simulink model "LyRStEnCtrl"  (R2018b)
settings: Solver=FixedStepDiscrete  StartTime=0.0  StopTime=10.0  FixedStep=0.01  RelTol=1e-3
undefined symbols (not defined in the file or in its folder): data, KeSMSw4SSecRwRtStLgrstUpwdDnwdOpenPos1_Val, SecRwRtStBkReclnEn_Clear, SecRwRtStBkReclnEn_Set, SecRwRtStFtrstEn_Clear, SecRwRtStFtrstEn_Set, SecRwRtStFwdBkwdEn_Clear, SecRwRtStFwdBkwdEn_Set, SecRwRtStHdrstFwdBkwdEn_Clear, SecRwRtStHdrstFwdBkwdEn_Set, SecRwRtStHdrstUpwdDnwdEn_Clear, SecRwRtStHdrstUpwdDnwdEn_Set, SecRwRtStLgrstInwdOtwdEn_Clear, SecRwRtStLgrstInwdOtwdEn_Set, SecRwRtStLgrstUpwdDnwdEn_Clear, SecRwRtStLgrstUpwdDnwdEn_Set
libraries: simulink x16
settings Model: ModifiedHistory="2023.11.16  V2.3.0 Issue 566045 全躺，vip，腿托打开增加前后位置"  Creator=sn2xws  LastModifiedBy=sn2xws
settings DataIOCC: SaveFormat=StructureWithTime
settings OptimizationCC: DefaultParameterBehavior=Inlined  EnhancedBackFolding=on  PassReuseOutputArgsAs=Individual arguments  ZeroExternalMemoryAtStartup=off  ZeroInternalMemoryAtStartup=off  OptimizeBlockOrder=speed  DifferentSizesBufferReuse=on  OptimizationCustomize=off
settings DebuggingCC: ParameterTunabilityLossMsg=error
settings ModelReferenceCC: ModelReferenceNumInstancesAllowed=Single
settings SFSimCC: MATLABDynamicMemAlloc=off
settings RTWCC: SystemTargetFile=autosar.tlc  GenCodeOnly=on  TemplateMakefile=ert_default_tmf  Description=AUTOSAR  GenerateReport=on  IncludeHyperlinkInReport=on  LaunchReport=on  GenerateTraceInfo=on  GenerateTraceReport=on  GenerateTraceReportSl=on  GenerateTraceReportSf=on  GenerateTraceReportEml=on
settings CodeAppCC: ForceParamTrailComments=on  IgnoreCustomStorageClasses=off  OperatorAnnotations=on  SimulinkDataObjDesc=on  SFDataObjDesc=on  InsertBlockDesc=on
settings STFCustomTargetCC: TargetLangStandard=C99 (ISO)  MultiwordLength=256  ParMdlRefBuildCompliant=on  CompOptLevelCompliant=on  IncludeMdlTerminateFcn=off  CombineOutputUpdateFcns=on  SuppressErrorStatus=on  ERTCustomFileBanners=on  SupportNonFinite=off  SupportComplex=off  SupportContinuousTime=off  SupportNonInlinedSFcns=off  RemoveResetFunc=on  MATLABClassNameForMDSCustomization=Simulink.SoftwareTarget.ERTCustomization  AutosarCompliant=on  UseToolchainInfoCompliant=on  LookupTableObjectStructAxisOrder=2,1,3,4,...  LUTObjectStructOrderEvenSpacing=Size,Table,Breakpoints  SystemTargetFile=autosar.tlc
settings ERTTargetCC: TargetLangStandard=C99 (ISO)  ConcurrentExecutionCompliant=off  IncludeMdlTerminateFcn=off  SuppressErrorStatus=on  SupportNonFinite=off  SupportComplex=off  ModelStepFunctionPrototypeControlCompliant=off  CPPClassGenCompliant=off  AutosarCompliant=on  LookupTableObjectStructAxisOrder=2,1,3,4,...  LUTObjectStructOrderEvenSpacing=Size,Table,Breakpoints  InlinedParameterPlacement=NonHierarchical  ERTCustomFileTemplate=example_file_process.tlc  ERTFilePackagingFormat=Compact

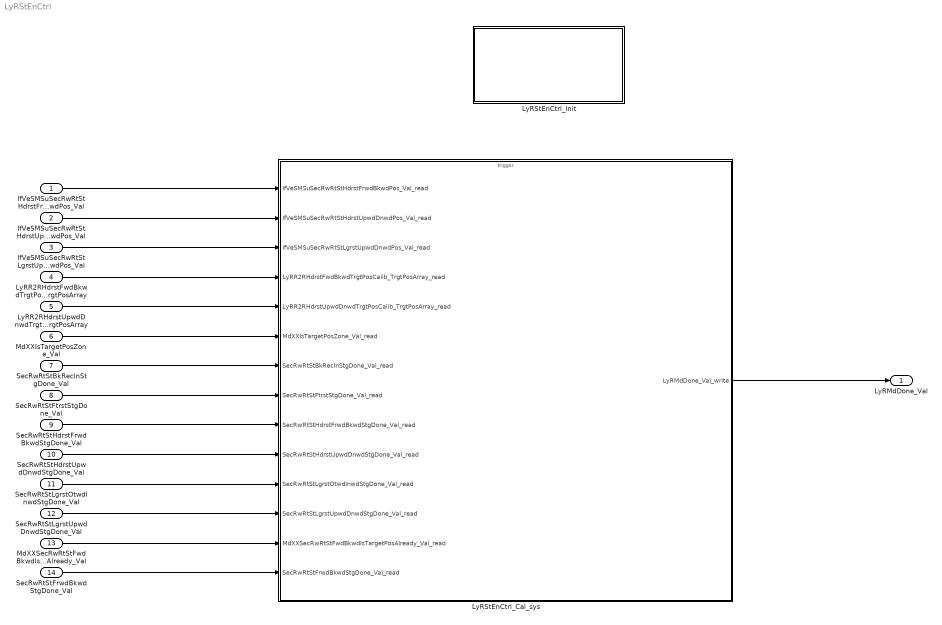
== system LyRStEnCtrl ==
  IfVeSMSuSecRwRtStHdrstFrwdBkwdPos_Val : Inport  OutDataTypeStr=uint16  PortDimensions=1
  IfVeSMSuSecRwRtStHdrstUpwdDnwdPos_Val : Inport  Port=2  OutDataTypeStr=uint16  PortDimensions=1
  IfVeSMSuSecRwRtStLgrstUpwdDnwdPos_Val : Inport  Port=3  OutDataTypeStr=uint16  PortDimensions=1
  LyRR2RHdrstFwdBkwdTrgtPosCalib_TrgtPosArray : Inport  Description=|  Port=4  OutDataTypeStr=uint16  PortDimensions=3
      | 0:Pos
      | 1:Max
      | 2:Min
  LyRR2RHdrstUpwdDnwdTrgtPosCalib_TrgtPosArray : Inport  Description=|  Port=5  OutDataTypeStr=uint16  PortDimensions=3
      | 0:Pos
      | 1:Max
      | 2:Min
  MdXXIsTargetPosZone_Val : Inport  Port=6  OutDataTypeStr=uint32  PortDimensions=1
  SecRwRtStBkReclnStgDone_Val : Inport  Port=7  OutDataTypeStr=boolean  PortDimensions=1
  SecRwRtStFtrstStgDone_Val : Inport  Port=8  OutDataTypeStr=boolean  PortDimensions=1
  SecRwRtStHdrstFrwdBkwdStgDone_Val : Inport  Port=9  OutDataTypeStr=boolean  PortDimensions=1
  SecRwRtStHdrstUpwdDnwdStgDone_Val : Inport  Port=10  OutDataTypeStr=boolean  PortDimensions=1
  SecRwRtStLgrstOtwdInwdStgDone_Val : Inport  Port=11  OutDataTypeStr=boolean  PortDimensions=1
  SecRwRtStLgrstUpwdDnwdStgDone_Val : Inport  Port=12  OutDataTypeStr=boolean  PortDimensions=1
  MdXXSecRwRtStFwdBkwdIsTargetPosAlready_Val : Inport  Port=13  OutDataTypeStr=uint32  PortDimensions=1
  SecRwRtStFrwdBkwdStgDone_Val : Inport  Port=14  OutDataTypeStr=boolean  PortDimensions=1
  LyRStEnCtrl_Cal_sys : Subsystem
  LyRStEnCtrl_Init : Subsystem
  LyRMdDone_Val : Outport  OutDataTypeStr=uint8  PortDimensions=1
  wires:
  IfVeSMSuSecRwRtStHdrstFrwdBkwdPos_Val/1 -> LyRStEnCtrl_Cal_sys/1(IfVeSMSuSecRwRtStHdrstFrwdBkwdPos_Val_read)
  IfVeSMSuSecRwRtStHdrstUpwdDnwdPos_Val/1 -> LyRStEnCtrl_Cal_sys/2(IfVeSMSuSecRwRtStHdrstUpwdDnwdPos_Val_read)
  IfVeSMSuSecRwRtStLgrstUpwdDnwdPos_Val/1 -> LyRStEnCtrl_Cal_sys/3(IfVeSMSuSecRwRtStLgrstUpwdDnwdPos_Val_read)
  LyRR2RHdrstFwdBkwdTrgtPosCalib_TrgtPosArray/1 -> LyRStEnCtrl_Cal_sys/4(LyRR2RHdrstFwdBkwdTrgtPosCalib_TrgtPosArray_read)
  LyRR2RHdrstUpwdDnwdTrgtPosCalib_TrgtPosArray/1 -> LyRStEnCtrl_Cal_sys/5(LyRR2RHdrstUpwdDnwdTrgtPosCalib_TrgtPosArray_read)
  MdXXIsTargetPosZone_Val/1 -> LyRStEnCtrl_Cal_sys/6(MdXXIsTargetPosZone_Val_read)
  SecRwRtStBkReclnStgDone_Val/1 -> LyRStEnCtrl_Cal_sys/7(SecRwRtStBkReclnStgDone_Val_read)
  SecRwRtStFtrstStgDone_Val/1 -> LyRStEnCtrl_Cal_sys/8(SecRwRtStFtrstStgDone_Val_read)
  SecRwRtStHdrstFrwdBkwdStgDone_Val/1 -> LyRStEnCtrl_Cal_sys/9(SecRwRtStHdrstFrwdBkwdStgDone_Val_read)
  SecRwRtStHdrstUpwdDnwdStgDone_Val/1 -> LyRStEnCtrl_Cal_sys/10(SecRwRtStHdrstUpwdDnwdStgDone_Val_read)
  SecRwRtStLgrstOtwdInwdStgDone_Val/1 -> LyRStEnCtrl_Cal_sys/11(SecRwRtStLgrstOtwdInwdStgDone_Val_read)
  SecRwRtStLgrstUpwdDnwdStgDone_Val/1 -> LyRStEnCtrl_Cal_sys/12(SecRwRtStLgrstUpwdDnwdStgDone_Val_read)
  LyRStEnCtrl_Cal_sys/1(LyRMdDone_Val_write) -> LyRMdDone_Val/1
  MdXXSecRwRtStFwdBkwdIsTargetPosAlready_Val/1 -> LyRStEnCtrl_Cal_sys/13(MdXXSecRwRtStFwdBkwdIsTargetPosAlready_Val_read)
  SecRwRtStFrwdBkwdStgDone_Val/1 -> LyRStEnCtrl_Cal_sys/14(SecRwRtStFrwdBkwdStgDone_Val_read)

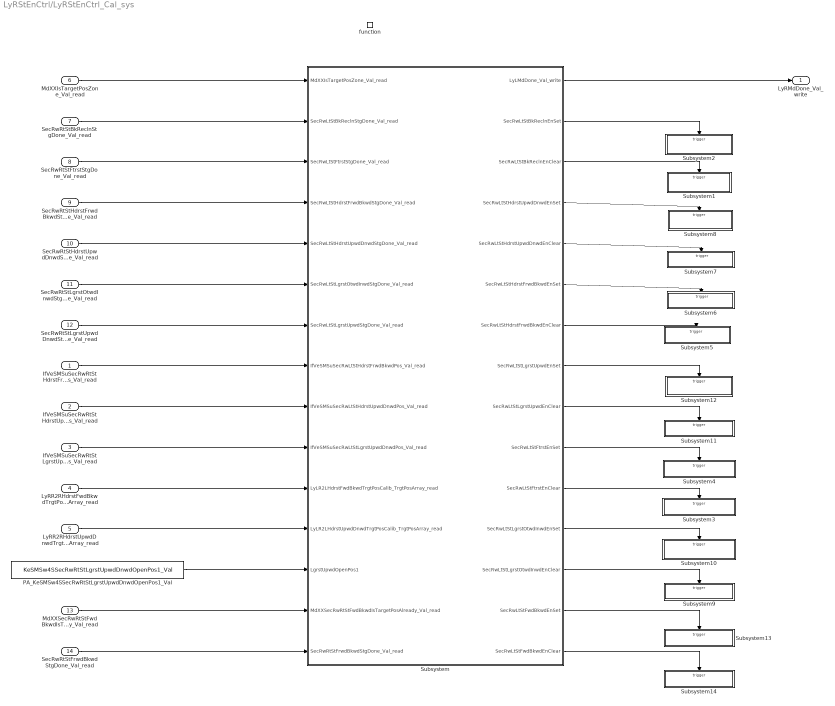
== system LyRStEnCtrl/LyRStEnCtrl_Cal_sys ==
  IfVeSMSuSecRwRtStHdrstFrwdBkwdPos_Val_read : Inport
  IfVeSMSuSecRwRtStHdrstUpwdDnwdPos_Val_read : Inport  Port=2
  IfVeSMSuSecRwRtStLgrstUpwdDnwdPos_Val_read : Inport  Port=3
  LyRR2RHdrstFwdBkwdTrgtPosCalib_TrgtPosArray_read : Inport  Port=4
  LyRR2RHdrstUpwdDnwdTrgtPosCalib_TrgtPosArray_read : Inport  Port=5
  MdXXIsTargetPosZone_Val_read : Inport  Port=6
  SecRwRtStBkReclnStgDone_Val_read : Inport  Port=7
  SecRwRtStFtrstStgDone_Val_read : Inport  Port=8
  SecRwRtStHdrstFrwdBkwdStgDone_Val_read : Inport  Port=9
  SecRwRtStHdrstUpwdDnwdStgDone_Val_read : Inport  Port=10
  SecRwRtStLgrstOtwdInwdStgDone_Val_read : Inport  Port=11
  SecRwRtStLgrstUpwdDnwdStgDone_Val_read : Inport  Port=12
  MdXXSecRwRtStFwdBkwdIsTargetPosAlready_Val_read : Inport  Port=13
  SecRwRtStFrwdBkwdStgDone_Val_read : Inport  Port=14
  function : TriggerPort  TriggerType=function-call  IsSimulinkFunction=on  FunctionName=LyRStEnCtrl_Cal  VariantControl=(inherit)
  PA_KeSMSw4SSecRwRtStLgrstUpwdDnwdOpenPos1_Val : Constant  Value=KeSMSw4SSecRwRtStLgrstUpwdDnwdOpenPos1_Val
  Subsystem : Subsystem
  Subsystem1 : Subsystem
  Subsystem10 : Subsystem
  Subsystem11 : Subsystem
  Subsystem12 : Subsystem
  Subsystem13 : Subsystem
  Subsystem14 : Subsystem
  Subsystem2 : Subsystem
  Subsystem3 : Subsystem
  Subsystem4 : Subsystem
  Subsystem5 : Subsystem
  Subsystem6 : Subsystem
  Subsystem7 : Subsystem
  Subsystem8 : Subsystem
  Subsystem9 : Subsystem
  LyRMdDone_Val_write : Outport
      settings: EnsureOutportIsVirtual=on
  wires:
  Subsystem/9(SecRwLtStLgrstUpwdEnClear) -> Subsystem11/Trigger
  Subsystem/12(SecRwLtStLgrstOtwdInwdEnSet) -> Subsystem10/Trigger
  Subsystem/13(SecRwLtStLgrstOtwdInwdEnClear) -> Subsystem9/Trigger
  Subsystem/10(SecRwLtStFtrstEnSet) -> Subsystem4/Trigger
  Subsystem/7(SecRwLtStHdrstFrwdBkwdEnClear) -> Subsystem5/Trigger
  Subsystem/8(SecRwLtStLgrstUpwdEnSet) -> Subsystem12/Trigger
  Subsystem/4(SecRwLtStHdrstUpwdDnwdEnSet) -> Subsystem8/Trigger
  Subsystem/3(SecRwLtStBkReclnEnClear) -> Subsystem1/Trigger
  Subsystem/6(SecRwLtStHdrstFrwdBkwdEnSet) -> Subsystem6/Trigger
  Subsystem/5(SecRwLtStHdrstUpwdDnwdEnClear) -> Subsystem7/Trigger
  Subsystem/2(SecRwLtStBkReclnEnSet) -> Subsystem2/Trigger
  Subsystem/11(SecRwLtStFtrstEnClear) -> Subsystem3/Trigger
  Subsystem/1(LyLMdDone_Val_write) -> LyRMdDone_Val_write/1
  PA_KeSMSw4SSecRwRtStLgrstUpwdDnwdOpenPos1_Val/1 -> Subsystem/13(LgrstUpwdOpenPos1)
  MdXXIsTargetPosZone_Val_read/1 -> Subsystem/1(MdXXIsTargetPosZone_Val_read)
  SecRwRtStBkReclnStgDone_Val_read/1 -> Subsystem/2(SecRwLtStBkReclnStgDone_Val_read)
  SecRwRtStFtrstStgDone_Val_read/1 -> Subsystem/3(SecRwLtStFtrstStgDone_Val_read)
  SecRwRtStHdrstFrwdBkwdStgDone_Val_read/1 -> Subsystem/4(SecRwLtStHdrstFrwdBkwdStgDone_Val_read)
  SecRwRtStHdrstUpwdDnwdStgDone_Val_read/1 -> Subsystem/5(SecRwLtStHdrstUpwdDnwdStgDone_Val_read)
  SecRwRtStLgrstOtwdInwdStgDone_Val_read/1 -> Subsystem/6(SecRwLtStLgrstOtwdInwdStgDone_Val_read)
  SecRwRtStLgrstUpwdDnwdStgDone_Val_read/1 -> Subsystem/7(SecRwLtStLgrstUpwdStgDone_Val_read)
  IfVeSMSuSecRwRtStHdrstFrwdBkwdPos_Val_read/1 -> Subsystem/8(IfVeSMSuSecRwLtStHdrstFrwdBkwdPos_Val_read)
  IfVeSMSuSecRwRtStHdrstUpwdDnwdPos_Val_read/1 -> Subsystem/9(IfVeSMSuSecRwLtStHdrstUpwdDnwdPos_Val_read)
  IfVeSMSuSecRwRtStLgrstUpwdDnwdPos_Val_read/1 -> Subsystem/10(IfVeSMSuSecRwLtStLgrstUpwdDnwdPos_Val_read)
  LyRR2RHdrstFwdBkwdTrgtPosCalib_TrgtPosArray_read/1 -> Subsystem/11(LyLR2LHdrstFwdBkwdTrgtPosCalib_TrgtPosArray_read)
  LyRR2RHdrstUpwdDnwdTrgtPosCalib_TrgtPosArray_read/1 -> Subsystem/12(LyLR2LHdrstUpwdDnwdTrgtPosCalib_TrgtPosArray_read)
  SecRwRtStFrwdBkwdStgDone_Val_read/1 -> Subsystem/15(SecRwRtStFrwdBkwdStgDone_Val_read)
  MdXXSecRwRtStFwdBkwdIsTargetPosAlready_Val_read/1 -> Subsystem/14(MdXXSecRwRtStFwdBkwdIsTargetPosAlready_Val_read)
  Subsystem/14(SecRwLtStFwdBkwdEnSet) -> Subsystem13/Trigger
  Subsystem/15(SecRwLtStFwdBkwdEnClear) -> Subsystem14/Trigger

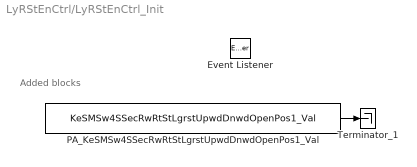
== system LyRStEnCtrl/LyRStEnCtrl_Init ==
  note: Added blocks
  Event Listener : EventListener  EventName=reset
  PA_KeSMSw4SSecRwRtStLgrstUpwdDnwdOpenPos1_Val : Constant  Value=KeSMSw4SSecRwRtStLgrstUpwdDnwdOpenPos1_Val
  Terminator_1 : Terminator
  wires:
  PA_KeSMSw4SSecRwRtStLgrstUpwdDnwdOpenPos1_Val/1 -> Terminator_1/1

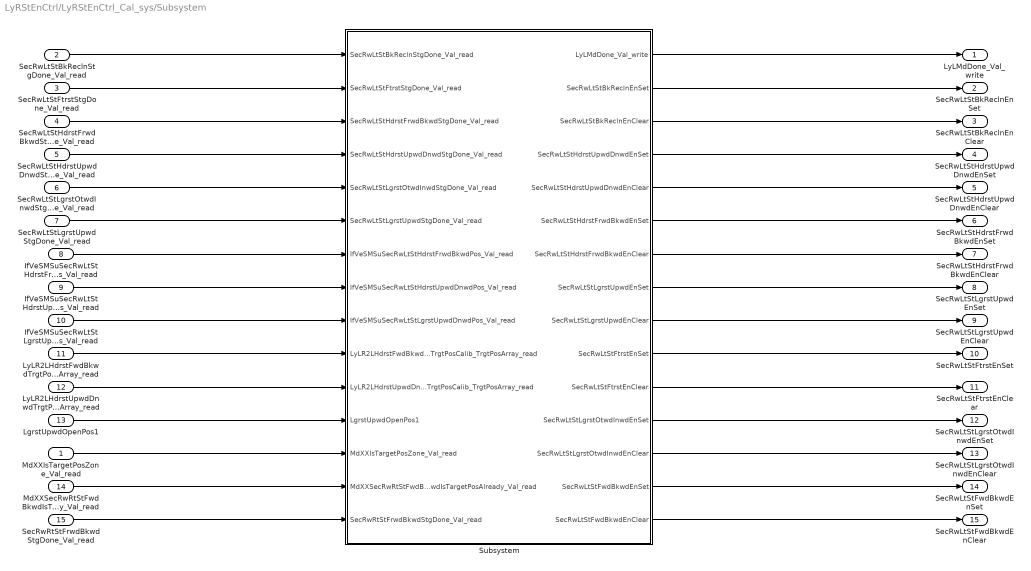
== system LyRStEnCtrl/LyRStEnCtrl_Cal_sys/Subsystem ==
  MdXXIsTargetPosZone_Val_read : Inport
  SecRwLtStBkReclnStgDone_Val_read : Inport  Port=2
  SecRwLtStFtrstStgDone_Val_read : Inport  Port=3
  SecRwLtStHdrstFrwdBkwdStgDone_Val_read : Inport  Port=4
  SecRwLtStHdrstUpwdDnwdStgDone_Val_read : Inport  Port=5
  SecRwLtStLgrstOtwdInwdStgDone_Val_read : Inport  Port=6
  SecRwLtStLgrstUpwdStgDone_Val_read : Inport  Port=7
  IfVeSMSuSecRwLtStHdrstFrwdBkwdPos_Val_read : Inport  Port=8
  IfVeSMSuSecRwLtStHdrstUpwdDnwdPos_Val_read : Inport  Port=9
  IfVeSMSuSecRwLtStLgrstUpwdDnwdPos_Val_read : Inport  Port=10
  LyLR2LHdrstFwdBkwdTrgtPosCalib_TrgtPosArray_read : Inport  Port=11
  LyLR2LHdrstUpwdDnwdTrgtPosCalib_TrgtPosArray_read : Inport  Port=12
  LgrstUpwdOpenPos1 : Inport  Port=13
  MdXXSecRwRtStFwdBkwdIsTargetPosAlready_Val_read : Inport  Port=14
  SecRwRtStFrwdBkwdStgDone_Val_read : Inport  Port=15
  Subsystem : Subsystem
  LyLMdDone_Val_write : Outport
      settings: EnsureOutportIsVirtual=on
  SecRwLtStBkReclnEnSet : Outport  Port=2
  SecRwLtStBkReclnEnClear : Outport  Port=3
  SecRwLtStHdrstUpwdDnwdEnSet : Outport  Port=4
  SecRwLtStHdrstUpwdDnwdEnClear : Outport  Port=5
  SecRwLtStHdrstFrwdBkwdEnSet : Outport  Port=6
  SecRwLtStHdrstFrwdBkwdEnClear : Outport  Port=7
  SecRwLtStLgrstUpwdEnSet : Outport  Port=8
  SecRwLtStLgrstUpwdEnClear : Outport  Port=9
  SecRwLtStFtrstEnSet : Outport  Port=10
  SecRwLtStFtrstEnClear : Outport  Port=11
  SecRwLtStLgrstOtwdInwdEnSet : Outport  Port=12
  SecRwLtStLgrstOtwdInwdEnClear : Outport  Port=13
  SecRwLtStFwdBkwdEnSet : Outport  Port=14
  SecRwLtStFwdBkwdEnClear : Outport  Port=15
  wires:
  SecRwLtStBkReclnStgDone_Val_read/1 -> Subsystem/1(SecRwLtStBkReclnStgDone_Val_read)
  SecRwLtStFtrstStgDone_Val_read/1 -> Subsystem/2(SecRwLtStFtrstStgDone_Val_read)
  SecRwLtStHdrstFrwdBkwdStgDone_Val_read/1 -> Subsystem/3(SecRwLtStHdrstFrwdBkwdStgDone_Val_read)
  SecRwLtStHdrstUpwdDnwdStgDone_Val_read/1 -> Subsystem/4(SecRwLtStHdrstUpwdDnwdStgDone_Val_read)
  SecRwLtStLgrstOtwdInwdStgDone_Val_read/1 -> Subsystem/5(SecRwLtStLgrstOtwdInwdStgDone_Val_read)
  SecRwLtStLgrstUpwdStgDone_Val_read/1 -> Subsystem/6(SecRwLtStLgrstUpwdStgDone_Val_read)
  IfVeSMSuSecRwLtStLgrstUpwdDnwdPos_Val_read/1 -> Subsystem/9(IfVeSMSuSecRwLtStLgrstUpwdDnwdPos_Val_read)
  IfVeSMSuSecRwLtStHdrstUpwdDnwdPos_Val_read/1 -> Subsystem/8(IfVeSMSuSecRwLtStHdrstUpwdDnwdPos_Val_read)
  LyLR2LHdrstUpwdDnwdTrgtPosCalib_TrgtPosArray_read/1 -> Subsystem/11(LyLR2LHdrstUpwdDnwdTrgtPosCalib_TrgtPosArray_read)
  LyLR2LHdrstFwdBkwdTrgtPosCalib_TrgtPosArray_read/1 -> Subsystem/10(LyLR2LHdrstFwdBkwdTrgtPosCalib_TrgtPosArray_read)
  IfVeSMSuSecRwLtStHdrstFrwdBkwdPos_Val_read/1 -> Subsystem/7(IfVeSMSuSecRwLtStHdrstFrwdBkwdPos_Val_read)
  MdXXIsTargetPosZone_Val_read/1 -> Subsystem/13(MdXXIsTargetPosZone_Val_read)
  LgrstUpwdOpenPos1/1 -> Subsystem/12(LgrstUpwdOpenPos1)
  Subsystem/1(LyLMdDone_Val_write) -> LyLMdDone_Val_write/1
  Subsystem/2(SecRwLtStBkReclnEnSet) -> SecRwLtStBkReclnEnSet/1
  Subsystem/3(SecRwLtStBkReclnEnClear) -> SecRwLtStBkReclnEnClear/1
  Subsystem/4(SecRwLtStHdrstUpwdDnwdEnSet) -> SecRwLtStHdrstUpwdDnwdEnSet/1
  Subsystem/5(SecRwLtStHdrstUpwdDnwdEnClear) -> SecRwLtStHdrstUpwdDnwdEnClear/1
  Subsystem/6(SecRwLtStHdrstFrwdBkwdEnSet) -> SecRwLtStHdrstFrwdBkwdEnSet/1
  Subsystem/7(SecRwLtStHdrstFrwdBkwdEnClear) -> SecRwLtStHdrstFrwdBkwdEnClear/1
  Subsystem/8(SecRwLtStLgrstUpwdEnSet) -> SecRwLtStLgrstUpwdEnSet/1
  Subsystem/9(SecRwLtStLgrstUpwdEnClear) -> SecRwLtStLgrstUpwdEnClear/1
  Subsystem/10(SecRwLtStFtrstEnSet) -> SecRwLtStFtrstEnSet/1
  Subsystem/11(SecRwLtStFtrstEnClear) -> SecRwLtStFtrstEnClear/1
  Subsystem/12(SecRwLtStLgrstOtwdInwdEnSet) -> SecRwLtStLgrstOtwdInwdEnSet/1
  Subsystem/13(SecRwLtStLgrstOtwdInwdEnClear) -> SecRwLtStLgrstOtwdInwdEnClear/1
  Subsystem/15(SecRwLtStFwdBkwdEnClear) -> SecRwLtStFwdBkwdEnClear/1
  Subsystem/14(SecRwLtStFwdBkwdEnSet) -> SecRwLtStFwdBkwdEnSet/1
  MdXXSecRwRtStFwdBkwdIsTargetPosAlready_Val_read/1 -> Subsystem/14(MdXXSecRwRtStFwdBkwdIsTargetPosAlready_Val_read)
  SecRwRtStFrwdBkwdStgDone_Val_read/1 -> Subsystem/15(SecRwRtStFrwdBkwdStgDone_Val_read)

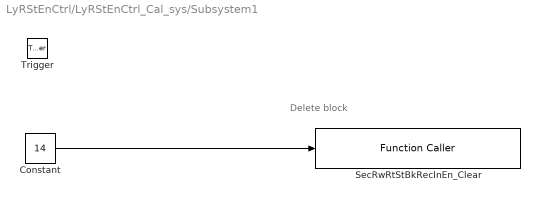
== system LyRStEnCtrl/LyRStEnCtrl_Cal_sys/Subsystem1 ==
  note: Delete block
  Trigger : TriggerPort  TriggerType=function-call  VariantControl=Variant  PortDimensions=1
  Constant : Constant  Value=14  OutDataTypeStr=uint8
  SecRwRtStBkReclnEn_Clear : FunctionCaller  FunctionPrototype=SecRwRtStBkReclnEn_Clear(data)  InputArgumentSpecifications=uint8(1)
  wires:
  Constant/1 -> SecRwRtStBkReclnEn_Clear/1

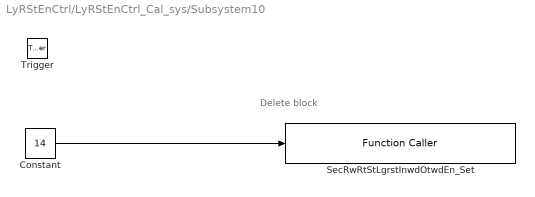
== system LyRStEnCtrl/LyRStEnCtrl_Cal_sys/Subsystem10 ==
  note: Delete block
  Trigger : TriggerPort  TriggerType=function-call  VariantControl=Variant  PortDimensions=1
  Constant : Constant  Value=14  OutDataTypeStr=uint8
  SecRwRtStLgrstInwdOtwdEn_Set : FunctionCaller  FunctionPrototype=SecRwRtStLgrstInwdOtwdEn_Set(data)  InputArgumentSpecifications=uint8(1)
  wires:
  Constant/1 -> SecRwRtStLgrstInwdOtwdEn_Set/1

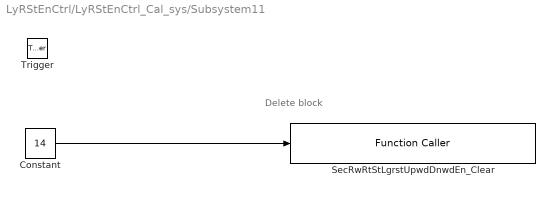
== system LyRStEnCtrl/LyRStEnCtrl_Cal_sys/Subsystem11 ==
  note: Delete block
  Trigger : TriggerPort  TriggerType=function-call  VariantControl=Variant  PortDimensions=1
  Constant : Constant  Value=14  OutDataTypeStr=uint8
  SecRwRtStLgrstUpwdDnwdEn_Clear : FunctionCaller  FunctionPrototype=SecRwRtStLgrstUpwdDnwdEn_Clear(data)  InputArgumentSpecifications=uint8(1)
  wires:
  Constant/1 -> SecRwRtStLgrstUpwdDnwdEn_Clear/1

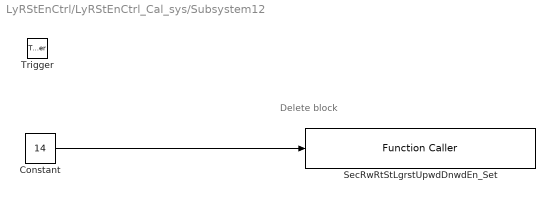
== system LyRStEnCtrl/LyRStEnCtrl_Cal_sys/Subsystem12 ==
  note: Delete block
  Trigger : TriggerPort  TriggerType=function-call  VariantControl=Variant  PortDimensions=1
  Constant : Constant  Value=14  OutDataTypeStr=uint8
  SecRwRtStLgrstUpwdDnwdEn_Set : FunctionCaller  FunctionPrototype=SecRwRtStLgrstUpwdDnwdEn_Set(data)  InputArgumentSpecifications=uint8(1)
  wires:
  Constant/1 -> SecRwRtStLgrstUpwdDnwdEn_Set/1

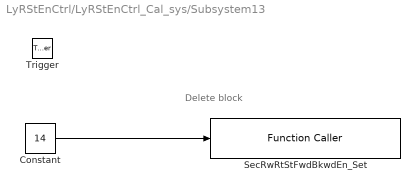
== system LyRStEnCtrl/LyRStEnCtrl_Cal_sys/Subsystem13 ==
  note: Delete block
  Trigger : TriggerPort  TriggerType=function-call  VariantControl=Variant  PortDimensions=1
  Constant : Constant  Value=14  OutDataTypeStr=uint8
  SecRwRtStFwdBkwdEn_Set : FunctionCaller  FunctionPrototype=SecRwRtStFwdBkwdEn_Set(data)  InputArgumentSpecifications=uint8(1)
  wires:
  Constant/1 -> SecRwRtStFwdBkwdEn_Set/1

== system LyRStEnCtrl/LyRStEnCtrl_Cal_sys/Subsystem14 ==
  note: Delete block
  Trigger : TriggerPort  TriggerType=function-call  VariantControl=Variant  PortDimensions=1
  Constant : Constant  Value=14  OutDataTypeStr=uint8
  SecRwRtStFwdBkwdEn_Clear : FunctionCaller  FunctionPrototype=SecRwRtStFwdBkwdEn_Clear(data)  InputArgumentSpecifications=uint8(1)
  wires:
  Constant/1 -> SecRwRtStFwdBkwdEn_Clear/1

== system LyRStEnCtrl/LyRStEnCtrl_Cal_sys/Subsystem2 ==
  note: Delete block
  Trigger : TriggerPort  TriggerType=function-call  VariantControl=Variant  PortDimensions=1
  Constant : Constant  Value=14  OutDataTypeStr=uint8
  SecRwRtStBkReclnEn_Set : FunctionCaller  FunctionPrototype=SecRwRtStBkReclnEn_Set(data)  InputArgumentSpecifications=uint8(1)
  wires:
  Constant/1 -> SecRwRtStBkReclnEn_Set/1

== system LyRStEnCtrl/LyRStEnCtrl_Cal_sys/Subsystem3 ==
  note: Delete block
  Trigger : TriggerPort  TriggerType=function-call  VariantControl=Variant  PortDimensions=1
  Constant : Constant  Value=14  OutDataTypeStr=uint8
  SecRwRtStFtrstEn_Clear : FunctionCaller  FunctionPrototype=SecRwRtStFtrstEn_Clear(data)  InputArgumentSpecifications=uint8(1)
  wires:
  Constant/1 -> SecRwRtStFtrstEn_Clear/1

== system LyRStEnCtrl/LyRStEnCtrl_Cal_sys/Subsystem4 ==
  note: Delete block
  Trigger : TriggerPort  TriggerType=function-call  VariantControl=Variant  PortDimensions=1
  Constant : Constant  Value=14  OutDataTypeStr=uint8
  SecRwRtStFtrstEn_Set : FunctionCaller  FunctionPrototype=SecRwRtStFtrstEn_Set(data)  InputArgumentSpecifications=uint8(1)
  wires:
  Constant/1 -> SecRwRtStFtrstEn_Set/1

== system LyRStEnCtrl/LyRStEnCtrl_Cal_sys/Subsystem5 ==
  note: Delete block
  Trigger : TriggerPort  TriggerType=function-call  VariantControl=Variant  PortDimensions=1
  Constant : Constant  Value=14  OutDataTypeStr=uint8
  SecRwRtStHdrstFwdBkwdEn_Clear : FunctionCaller  FunctionPrototype=SecRwRtStHdrstFwdBkwdEn_Clear(data)  InputArgumentSpecifications=uint8(1)
  wires:
  Constant/1 -> SecRwRtStHdrstFwdBkwdEn_Clear/1

== system LyRStEnCtrl/LyRStEnCtrl_Cal_sys/Subsystem6 ==
  note: Delete block
  Trigger : TriggerPort  TriggerType=function-call  VariantControl=Variant  PortDimensions=1
  Constant : Constant  Value=14  OutDataTypeStr=uint8
  SecRwRtStHdrstFwdBkwdEn_Set : FunctionCaller  FunctionPrototype=SecRwRtStHdrstFwdBkwdEn_Set(data)  InputArgumentSpecifications=uint8(1)
  wires:
  Constant/1 -> SecRwRtStHdrstFwdBkwdEn_Set/1

== system LyRStEnCtrl/LyRStEnCtrl_Cal_sys/Subsystem7 ==
  note: Delete block
  Trigger : TriggerPort  TriggerType=function-call  VariantControl=Variant  PortDimensions=1
  Constant : Constant  Value=14  OutDataTypeStr=uint8
  SecRwRtStHdrstUpwdDnwdEn_Clear : FunctionCaller  FunctionPrototype=SecRwRtStHdrstUpwdDnwdEn_Clear(data)  InputArgumentSpecifications=uint8(1)
  wires:
  Constant/1 -> SecRwRtStHdrstUpwdDnwdEn_Clear/1

== system LyRStEnCtrl/LyRStEnCtrl_Cal_sys/Subsystem8 ==
  note: Delete block
  Trigger : TriggerPort  TriggerType=function-call  VariantControl=Variant  PortDimensions=1
  Constant : Constant  Value=14  OutDataTypeStr=uint8
  SecRwRtStHdrstUpwdDnwdEn_Set : FunctionCaller  FunctionPrototype=SecRwRtStHdrstUpwdDnwdEn_Set(data)  InputArgumentSpecifications=uint8(1)
  wires:
  Constant/1 -> SecRwRtStHdrstUpwdDnwdEn_Set/1

== system LyRStEnCtrl/LyRStEnCtrl_Cal_sys/Subsystem9 ==
  note: Delete block
  Trigger : TriggerPort  TriggerType=function-call  VariantControl=Variant  PortDimensions=1
  Constant : Constant  Value=14  OutDataTypeStr=uint8
  SecRwRtStLgrstInwdOtwdEn_Clear : FunctionCaller  FunctionPrototype=SecRwRtStLgrstInwdOtwdEn_Clear(data)  InputArgumentSpecifications=uint8(1)
  wires:
  Constant/1 -> SecRwRtStLgrstInwdOtwdEn_Clear/1

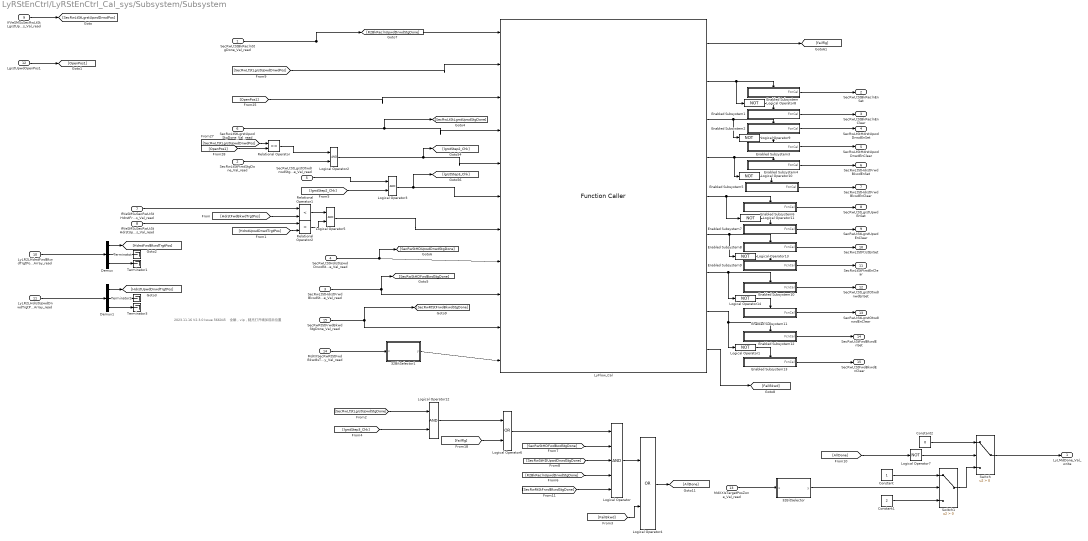
== system LyRStEnCtrl/LyRStEnCtrl_Cal_sys/Subsystem/Subsystem ==
  note: 2023.11.16 V2.3.0 Issue 566045 全躺，vip，腿托打开增加前后位置
  SecRwLtStBkReclnStgDone_Val_read : Inport
  SecRwLtStFtrstStgDone_Val_read : Inport  Port=2
  SecRwLtStHdrstFrwdBkwdStgDone_Val_read : Inport  Port=3
  SecRwLtStHdrstUpwdDnwdStgDone_Val_read : Inport  Port=4
  SecRwLtStLgrstOtwdInwdStgDone_Val_read : Inport  Port=5
  SecRwLtStLgrstUpwdStgDone_Val_read : Inport  Port=6
  IfVeSMSuSecRwLtStHdrstFrwdBkwdPos_Val_read : Inport  Port=7
  IfVeSMSuSecRwLtStHdrstUpwdDnwdPos_Val_read : Inport  Port=8
  IfVeSMSuSecRwLtStLgrstUpwdDnwdPos_Val_read : Inport  Port=9
  LyLR2LHdrstFwdBkwdTrgtPosCalib_TrgtPosArray_read : Inport  Port=10
  LyLR2LHdrstUpwdDnwdTrgtPosCalib_TrgtPosArray_read : Inport  Port=11
  LgrstUpwdOpenPos1 : Inport  Port=12
  MdXXIsTargetPosZone_Val_read : Inport  Port=13
  MdXXSecRwRtStFwdBkwdIsTargetPosAlready_Val_read : Inport  Port=14
  SecRwRtStFrwdBkwdStgDone_Val_read : Inport  Port=15
  32BitSelector : Subsystem  mask(32 Bit Selector){BitNum=14}
      mask prompts: BitNum "Select Bit Number"
      mask help: Allows selection of a particular bit (0-31) out of a packed word up to 32 bits long. Output will be true if the bit number selected via the mask parameter is equal to one.
      mask TypeOptions BitNum: 0 | 1 | 2 | 3 | 4 | 5 | 6 | 7 | 8 | 9 | 10 | 11 | 12 | 13 | 14 | 15 | 16 | 17 | 18 | 19 | 20 | 21 | 22 | 23 | 24 | 25 | 26 | 27 | 28 | 29 | 30 | 31
      mask Display:
      | text(0.5, 0.8,'BIT','horizontalAlignment','center')
      | text(0.5, 0.5,'SELECTOR','horizontalAlignment','center')
      | text(0.5, 0.2,['-- Bit ',char(get_param(gcb,'BitNum')),' --'],'horizontalAlignment','center')
  32BitSelector1 : Subsystem  mask(32 Bit Selector){BitNum=14}
      mask prompts: BitNum "Select Bit Number"
      mask help: Allows selection of a particular bit (0-31) out of a packed word up to 32 bits long. Output will be true if the bit number selected via the mask parameter is equal to one.
      mask TypeOptions BitNum: 0 | 1 | 2 | 3 | 4 | 5 | 6 | 7 | 8 | 9 | 10 | 11 | 12 | 13 | 14 | 15 | 16 | 17 | 18 | 19 | 20 | 21 | 22 | 23 | 24 | 25 | 26 | 27 | 28 | 29 | 30 | 31
      mask Display:
      | text(0.5, 0.8,'BIT','horizontalAlignment','center')
      | text(0.5, 0.5,'SELECTOR','horizontalAlignment','center')
      | text(0.5, 0.2,['-- Bit ',char(get_param(gcb,'BitNum')),' --'],'horizontalAlignment','center')
  Constant : Constant  OutDataTypeStr=uint8
  Constant1 : Constant  Value=2  OutDataTypeStr=uint8
  Constant2 : Constant  Value=0  OutDataTypeStr=uint8
  Demux : Demux  Outputs=3
  Demux1 : Demux  Outputs=3
  Enabled Subsystem : Subsystem  TreatAsAtomicUnit=on
  Enabled Subsystem1 : Subsystem  TreatAsAtomicUnit=on
  Enabled Subsystem10 : Subsystem  TreatAsAtomicUnit=on
  Enabled Subsystem11 : Subsystem  TreatAsAtomicUnit=on
  Enabled Subsystem12 : Subsystem  TreatAsAtomicUnit=on
  Enabled Subsystem13 : Subsystem  TreatAsAtomicUnit=on
  Enabled Subsystem2 : Subsystem  TreatAsAtomicUnit=on
  Enabled Subsystem3 : Subsystem  TreatAsAtomicUnit=on
  Enabled Subsystem4 : Subsystem  TreatAsAtomicUnit=on
  Enabled Subsystem5 : Subsystem  TreatAsAtomicUnit=on
  Enabled Subsystem6 : Subsystem  TreatAsAtomicUnit=on
  Enabled Subsystem7 : Subsystem  TreatAsAtomicUnit=on
  Enabled Subsystem8 : Subsystem  TreatAsAtomicUnit=on
  Enabled Subsystem9 : Subsystem  TreatAsAtomicUnit=on
  Logical Operator : Logic  Inputs=5  AllPortsSameDT=off  OutDataTypeStr=boolean
  Logical Operator{1,7..11,13..14} (8 alike) : Logic  Operator=NOT  AllPortsSameDT=off  OutDataTypeStr=boolean
  Logical Operator{2..3,5,12} (4 alike) : Logic  AllPortsSameDT=off  OutDataTypeStr=boolean
  Logical Operator4 : Logic  Operator=OR  AllPortsSameDT=off  OutDataTypeStr=boolean
  Logical Operator6 : Logic  Operator=OR  AllPortsSameDT=off  OutDataTypeStr=boolean
  LyFlow_Cal : FunctionCaller  FunctionPrototype=[Failflg,BkReclnEn,HdrstUpwdEn,HdrstFrwdEn,LgrstUpwdDnwdEn,FtrstEn,LgrstInwdOtwdEn,FwdBkwdEn,FailBkwd] = LyFlow_Cal(BkReclnStgDone,LgrstUpwdDnwdPos,LgrstUpwdDnwdOpenPos1,LgrstUpwdStgDone,FtrstStgDone,LgrstInwdStgDone,Chkhdflg,HdrstUpwdDnwdStgDone,HdrstFrwdBkwdStgDone,FwdBkwdStgDone,FwdBkwdIsPosAlready)  InputArgumentSpecifications=boolean(true), uint16(1), uint16(1), boolean(true), boolean(true), boolean(true), boolean(true), boolean(true), boolean(true), boolean(true), boolean(true)  OutputArgumentSpecifications=boolean(true), boolean(true), boolean(true), boolean(true), boolean(true), boolean(true), boolean(true), boolean(true), boolean(true)
  Relational Operator : RelationalOperator  OutDataTypeStr=boolean  RndMeth=Simplest
  Relational Operator1 : RelationalOperator  Operator=<  OutDataTypeStr=boolean  RndMeth=Simplest
  Relational Operator2 : RelationalOperator  Operator=<  OutDataTypeStr=boolean  RndMeth=Simplest
  Switch : Switch  Criteria=u2 > Threshold
  Switch1 : Switch  Criteria=u2 > Threshold
  Terminator{,1..3} (4 alike) : Terminator
  LyLMdDone_Val_write : Outport
      settings: EnsureOutportIsVirtual=on
  SecRwLtStBkReclnEnSet : Outport  Port=2
  SecRwLtStBkReclnEnClear : Outport  Port=3
  SecRwLtStHdrstUpwdDnwdEnSet : Outport  Port=4
  SecRwLtStHdrstUpwdDnwdEnClear : Outport  Port=5
  SecRwLtStHdrstFrwdBkwdEnSet : Outport  Port=6
  SecRwLtStHdrstFrwdBkwdEnClear : Outport  Port=7
  SecRwLtStLgrstUpwdEnSet : Outport  Port=8
  SecRwLtStLgrstUpwdEnClear : Outport  Port=9
  SecRwLtStFtrstEnSet : Outport  Port=10
  SecRwLtStFtrstEnClear : Outport  Port=11
  SecRwLtStLgrstOtwdInwdEnSet : Outport  Port=12
  SecRwLtStLgrstOtwdInwdEnClear : Outport  Port=13
  SecRwLtStFwdBkwdEnSet : Outport  Port=14
  SecRwLtStFwdBkwdEnClear : Outport  Port=15
  wires:
  [SecRwLtStLgrstUpwdDnwdPos] -> Relational Operator/1
  Relational Operator/1 -> Logical Operator2/1
  [OpenPos1] -> LyFlow_Cal/3
  Logical Operator2/1 -> LyFlow_Cal/5, [lgrstStep2_Chk]
  IfVeSMSuSecRwLtStHdrstFrwdBkwdPos_Val_read/1 -> Relational Operator1/1
  [OpenPos1] -> Relational Operator/2
  Logical Operator3/1 -> LyFlow_Cal/6, [lgrstStep3_Chk]
  SecRwLtStLgrstUpwdStgDone_Val_read/1 -> LyFlow_Cal/4, [SecRwLtStLgrstUpwdStgDone]
  SecRwLtStFtrstStgDone_Val_read/1 -> Logical Operator2/2
  SecRwLtStBkReclnStgDone_Val_read/1 -> [R2BkReclnUpwdDnwdStgDone], LyFlow_Cal/1
  SecRwLtStLgrstOtwdInwdStgDone_Val_read/1 -> Logical Operator3/1
  Relational Operator2/1 -> Logical Operator5/2
  Relational Operator1/1 -> Logical Operator5/1
  SecRwLtStHdrstFrwdBkwdStgDone_Val_read/1 -> [SecRwStHDFwdBwdStgDone], LyFlow_Cal/9
  LyFlow_Cal/1 -> [failflg]
  Logical Operator5/1 -> LyFlow_Cal/7
  [lgrstStep2_Chk] -> Logical Operator3/2
  IfVeSMSuSecRwLtStHdrstUpwdDnwdPos_Val_read/1 -> Relational Operator2/1
  SecRwLtStHdrstUpwdDnwdStgDone_Val_read/1 -> [SecRwStHDUpwdDnwdStgDone], LyFlow_Cal/8
  [SecRwLtStLgrstUpwdDnwdPos] -> LyFlow_Cal/2
  IfVeSMSuSecRwLtStLgrstUpwdDnwdPos_Val_read/1 -> [SecRwLtStLgrstUpwdDnwdPos]
  LgrstUpwdOpenPos1/1 -> [OpenPos1]
  LyLR2LHdrstFwdBkwdTrgtPosCalib_TrgtPosArray_read/1 -> Demux/1
  Demux/1 -> [HdrstFwdBkwdTrgtPos]
  Demux1/1 -> [HdrstUpwdDnwdTrgtPos]
  LyLR2LHdrstUpwdDnwdTrgtPosCalib_TrgtPosArray_read/1 -> Demux1/1
  Demux/2 -> Terminator/1
  Demux/3 -> Terminator1/1
  Demux1/3 -> Terminator3/1
  Demux1/2 -> Terminator2/1
  [HdrstFwdBkwdTrgtPos] -> Relational Operator1/2
  [HdrstUpwdDnwdTrgtPos] -> Relational Operator2/2
  [SecRwLtStLgrstUpwdStgDone] -> Logical Operator12/1
  [lgrstStep3_Chk] -> Logical Operator12/2
  [failflg] -> Logical Operator6/2
  Logical Operator12/1 -> Logical Operator6/1
  [SecRwStHDUpwdDnwdStgDone] -> Logical Operator/3
  Logical Operator6/1 -> Logical Operator/1
  [R2BkReclnUpwdDnwdStgDone] -> Logical Operator/4
  [SecRwStHDFwdBwdStgDone] -> Logical Operator/2
  Switch1/1 -> Switch/3
  Switch/1 -> LyLMdDone_Val_write/1
  MdXXIsTargetPosZone_Val_read/1 -> 32BitSelector/1(x)
  Enabled Subsystem7/1(FcnCal) -> SecRwLtStLgrstUpwdEnClear/1
  Enabled Subsystem11/1(FcnCal) -> SecRwLtStLgrstOtwdInwdEnClear/1
  LyFlow_Cal/5 -> Enabled Subsystem6/Enable, Logical Operator11/1
  LyFlow_Cal/6 -> Logical Operator13/1, Enabled Subsystem8/Enable
  Enabled Subsystem10/1(FcnCal) -> SecRwLtStLgrstOtwdInwdEnSet/1
  Enabled Subsystem3/1(FcnCal) -> SecRwLtStHdrstUpwdDnwdEnClear/1
  Enabled Subsystem8/1(FcnCal) -> SecRwLtStFtrstEnSet/1
  Enabled Subsystem2/1(FcnCal) -> SecRwLtStHdrstUpwdDnwdEnSet/1
  Enabled Subsystem4/1(FcnCal) -> SecRwLtStHdrstFrwdBkwdEnSet/1
  Enabled Subsystem5/1(FcnCal) -> SecRwLtStHdrstFrwdBkwdEnClear/1
  Logical Operator13/1 -> Enabled Subsystem9/Enable
  Enabled Subsystem1/1(FcnCal) -> SecRwLtStBkReclnEnClear/1
  Logical Operator8/1 -> Enabled Subsystem1/Enable
  Enabled Subsystem6/1(FcnCal) -> SecRwLtStLgrstUpwdEnSet/1
  Enabled Subsystem/1(FcnCal) -> SecRwLtStBkReclnEnSet/1
  LyFlow_Cal/3 -> Logical Operator9/1, Enabled Subsystem2/Enable
  Enabled Subsystem9/1(FcnCal) -> SecRwLtStFtrstEnClear/1
  Logical Operator11/1 -> Enabled Subsystem7/Enable
  LyFlow_Cal/7 -> Enabled Subsystem10/Enable, Logical Operator14/1
  Logical Operator10/1 -> Enabled Subsystem5/Enable
  Logical Operator9/1 -> Enabled Subsystem3/Enable
  LyFlow_Cal/2 -> Logical Operator8/1, Enabled Subsystem/Enable
  LyFlow_Cal/4 -> Logical Operator10/1, Enabled Subsystem4/Enable
  Logical Operator14/1 -> Enabled Subsystem11/Enable
  Constant2/1 -> Switch/1
  Constant1/1 -> Switch1/3
  Constant/1 -> Switch1/1
  [AllDone] -> Logical Operator7/1
  Logical Operator7/1 -> Switch/2
  32BitSelector/1(y) -> Switch1/2
  Logical Operator1/1 -> Enabled Subsystem13/Enable
  LyFlow_Cal/8 -> Logical Operator1/1, Enabled Subsystem12/Enable
  Enabled Subsystem12/1(FcnCal) -> SecRwLtStFwdBkwdEnSet/1
  Enabled Subsystem13/1(FcnCal) -> SecRwLtStFwdBkwdEnClear/1
  LyFlow_Cal/9 -> [FailBkwd]
  Logical Operator/1 -> Logical Operator4/1
  [FailBkwd] -> Logical Operator4/2
  Logical Operator4/1 -> [AllDone]
  SecRwRtStFrwdBkwdStgDone_Val_read/1 -> [SecRwRtStFrwdBkwdStgDone], LyFlow_Cal/10
  MdXXSecRwRtStFwdBkwdIsTargetPosAlready_Val_read/1 -> 32BitSelector1/1(x)
  32BitSelector1/1(y) -> LyFlow_Cal/11
  [SecRwRtStFrwdBkwdStgDone] -> Logical Operator/5

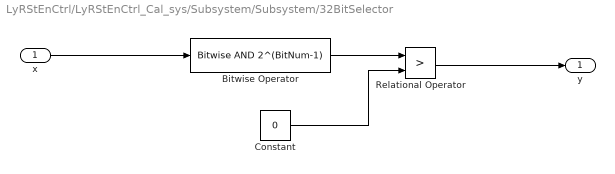
== system LyRStEnCtrl/LyRStEnCtrl_Cal_sys/Subsystem/Subsystem/32BitSelector ==
  x : Inport
  Bitwise Operator : simulink/Logic and Bit Operations/Bitwise Operator  logicop=AND  UseBitMask=on  BitMask=2^(BitNum-1)  BitMaskRealWorld=Stored Integer
  Constant : Constant  Value=0  OutDataTypeStr=uint32
  Relational Operator : RelationalOperator  Operator=>  OutDataTypeStr=boolean  RndMeth=Simplest
  y : Outport
  wires:
  Relational Operator/1 -> y/1
  Constant/1 -> Relational Operator/2
  x/1 -> Bitwise Operator/1
  Bitwise Operator/1 -> Relational Operator/1

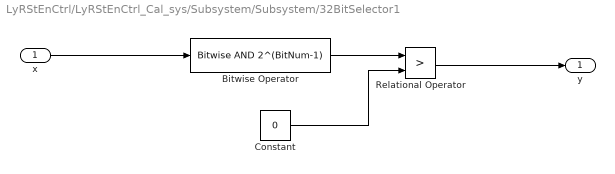
== system LyRStEnCtrl/LyRStEnCtrl_Cal_sys/Subsystem/Subsystem/32BitSelector1 ==
  x : Inport
  Bitwise Operator : simulink/Logic and Bit Operations/Bitwise Operator  logicop=AND  UseBitMask=on  BitMask=2^(BitNum-1)  BitMaskRealWorld=Stored Integer
  Constant : Constant  Value=0  OutDataTypeStr=uint32
  Relational Operator : RelationalOperator  Operator=>  OutDataTypeStr=boolean  RndMeth=Simplest
  y : Outport
  wires:
  Bitwise Operator/1 -> Relational Operator/1
  x/1 -> Bitwise Operator/1
  Constant/1 -> Relational Operator/2
  Relational Operator/1 -> y/1

== system LyRStEnCtrl/LyRStEnCtrl_Cal_sys/Subsystem/Subsystem/Enabled Subsystem ==
  Enable : EnablePort
  Function-Call Generator : simulink/Ports & Subsystems/Function-Call Generator  sample_time=-1  numberOfIterations=1
  FcnCal : Outport
  wires:
  Function-Call Generator/1 -> FcnCal/1

== system LyRStEnCtrl/LyRStEnCtrl_Cal_sys/Subsystem/Subsystem/Enabled Subsystem1 ==
  Enable : EnablePort
  Function-Call Generator : simulink/Ports & Subsystems/Function-Call Generator  sample_time=-1  numberOfIterations=1
  FcnCal : Outport
  wires:
  Function-Call Generator/1 -> FcnCal/1

== system LyRStEnCtrl/LyRStEnCtrl_Cal_sys/Subsystem/Subsystem/Enabled Subsystem10 ==
  Enable : EnablePort
  Function-Call Generator : simulink/Ports & Subsystems/Function-Call Generator  sample_time=-1  numberOfIterations=1
  FcnCal : Outport
  wires:
  Function-Call Generator/1 -> FcnCal/1

== system LyRStEnCtrl/LyRStEnCtrl_Cal_sys/Subsystem/Subsystem/Enabled Subsystem11 ==
  Enable : EnablePort
  Function-Call Generator : simulink/Ports & Subsystems/Function-Call Generator  sample_time=-1  numberOfIterations=1
  FcnCal : Outport
  wires:
  Function-Call Generator/1 -> FcnCal/1

== system LyRStEnCtrl/LyRStEnCtrl_Cal_sys/Subsystem/Subsystem/Enabled Subsystem12 ==
  Enable : EnablePort
  Function-Call Generator : simulink/Ports & Subsystems/Function-Call Generator  sample_time=-1  numberOfIterations=1
  FcnCal : Outport
  wires:
  Function-Call Generator/1 -> FcnCal/1

== system LyRStEnCtrl/LyRStEnCtrl_Cal_sys/Subsystem/Subsystem/Enabled Subsystem13 ==
  Enable : EnablePort
  Function-Call Generator : simulink/Ports & Subsystems/Function-Call Generator  sample_time=-1  numberOfIterations=1
  FcnCal : Outport
  wires:
  Function-Call Generator/1 -> FcnCal/1

== system LyRStEnCtrl/LyRStEnCtrl_Cal_sys/Subsystem/Subsystem/Enabled Subsystem2 ==
  Enable : EnablePort
  Function-Call Generator : simulink/Ports & Subsystems/Function-Call Generator  sample_time=-1  numberOfIterations=1
  FcnCal : Outport
  wires:
  Function-Call Generator/1 -> FcnCal/1

== system LyRStEnCtrl/LyRStEnCtrl_Cal_sys/Subsystem/Subsystem/Enabled Subsystem3 ==
  Enable : EnablePort
  Function-Call Generator : simulink/Ports & Subsystems/Function-Call Generator  sample_time=-1  numberOfIterations=1
  FcnCal : Outport
  wires:
  Function-Call Generator/1 -> FcnCal/1

== system LyRStEnCtrl/LyRStEnCtrl_Cal_sys/Subsystem/Subsystem/Enabled Subsystem4 ==
  Enable : EnablePort
  Function-Call Generator : simulink/Ports & Subsystems/Function-Call Generator  sample_time=-1  numberOfIterations=1
  FcnCal : Outport
  wires:
  Function-Call Generator/1 -> FcnCal/1

== system LyRStEnCtrl/LyRStEnCtrl_Cal_sys/Subsystem/Subsystem/Enabled Subsystem5 ==
  Enable : EnablePort
  Function-Call Generator : simulink/Ports & Subsystems/Function-Call Generator  sample_time=-1  numberOfIterations=1
  FcnCal : Outport
  wires:
  Function-Call Generator/1 -> FcnCal/1

== system LyRStEnCtrl/LyRStEnCtrl_Cal_sys/Subsystem/Subsystem/Enabled Subsystem6 ==
  Enable : EnablePort
  Function-Call Generator : simulink/Ports & Subsystems/Function-Call Generator  sample_time=-1  numberOfIterations=1
  FcnCal : Outport
  wires:
  Function-Call Generator/1 -> FcnCal/1

== system LyRStEnCtrl/LyRStEnCtrl_Cal_sys/Subsystem/Subsystem/Enabled Subsystem7 ==
  Enable : EnablePort
  Function-Call Generator : simulink/Ports & Subsystems/Function-Call Generator  sample_time=-1  numberOfIterations=1
  FcnCal : Outport
  wires:
  Function-Call Generator/1 -> FcnCal/1

== system LyRStEnCtrl/LyRStEnCtrl_Cal_sys/Subsystem/Subsystem/Enabled Subsystem8 ==
  Enable : EnablePort
  Function-Call Generator : simulink/Ports & Subsystems/Function-Call Generator  sample_time=-1  numberOfIterations=1
  FcnCal : Outport
  wires:
  Function-Call Generator/1 -> FcnCal/1

== system LyRStEnCtrl/LyRStEnCtrl_Cal_sys/Subsystem/Subsystem/Enabled Subsystem9 ==
  Enable : EnablePort
  Function-Call Generator : simulink/Ports & Subsystems/Function-Call Generator  sample_time=-1  numberOfIterations=1
  FcnCal : Outport
  wires:
  Function-Call Generator/1 -> FcnCal/1
